simulink model "vehicleVariantsLabel"  (R2020a)
settings: Solver=VariableStepAuto  StartTime=0.0  StopTime=30  FixedStep=Ts  RelTol=1e-3
model workspace: external: MAT-File data.mat (data not in the file)
values from neighbouring files (symbols this model uses):
  fsw = 9000    [data.mat]
  ID_MAP = [-123.486133396 -123.486133396 -123.486133396 -123.486133396 -123.486133396 -123.486133396 -123.486133396 -123.486133396 -123.486133396 -123.486133396 -123.486133396 -123.486133396 ... (280623 elements, 161x83x21)]    [data.mat]
  IQ_MAP = [-339.521551914 -339.521551914 -339.521551914 -339.521551914 -339.521551914 -339.521551914 -339.521551914 -339.521551914 -339.521551914 -339.521551914 -339.521551914 -339.521551914 ... (280623 elements, 161x83x21)]    [data.mat]
  Ki_v = 70    [data.mat]
  Kp_v = 150    [data.mat]
  Ld = 0.00024368    [data.mat]
  Lq = 0.00029758    [data.mat]
  motorOn = 1    [data.mat]
  p = 8    [data.mat]
  Pmax = 35000    [data.mat]
  psim = 0.04366    [data.mat]
  recumax = -50    [data.mat]
  RPM_VECT = [0 100 200 300 400 500 600 700 800 900 1000 1100 ... (161 elements, 1x161)]    [data.mat]
  rreifen = 0.3237    [data.mat]
  Tmax = 205    [data.mat]
  TQ_VECT = [-205 -200 -195 -190 -185 -180 -175 -170 -165 -160 -155 -150 ... (83 elements, 1x83)]    [data.mat]
  Ts = 5e-05    [data.mat]
  Tsi = 5e-05    [data.mat]
  Tso = 0.0005    [data.mat]
  VDC_VECT = [300 305 310 315 320 325 330 335 340 345 350 355 ... (21 elements, 1x21)]    [data.mat]
  Vnom = 325    [data.mat]
undefined symbols (not defined in the file or in its folder): DiscIntNeverNeededParam, sigbuilder_block
libraries: fl_lib x42, nesl_utility x20, ee_lib x8, simulink x2, eeTransforms x2, eeDiscretePi x1, eePmsmCurrentController x1, eePwmGeneratorTwoLevel x1
(part 1 of 2)
settings Model: SimulationMode=accelerator  OrderedModelArguments=off  Creator=ftutschk  LastModifiedBy=ftutschk
settings DataIOCC: SaveOutput=off  DSMLogging=off  SaveTime=off  ReturnWorkspaceOutputs=off
settings DebuggingCC: ArithmeticOperatorsInVariantConditions=warning
settings SFSimCC: SimUseLocalCustomCode=off  CustomCodeUndefinedFunction=UseInterfaceOnly
settings RTWCC: RTWUseLocalCustomCode=off

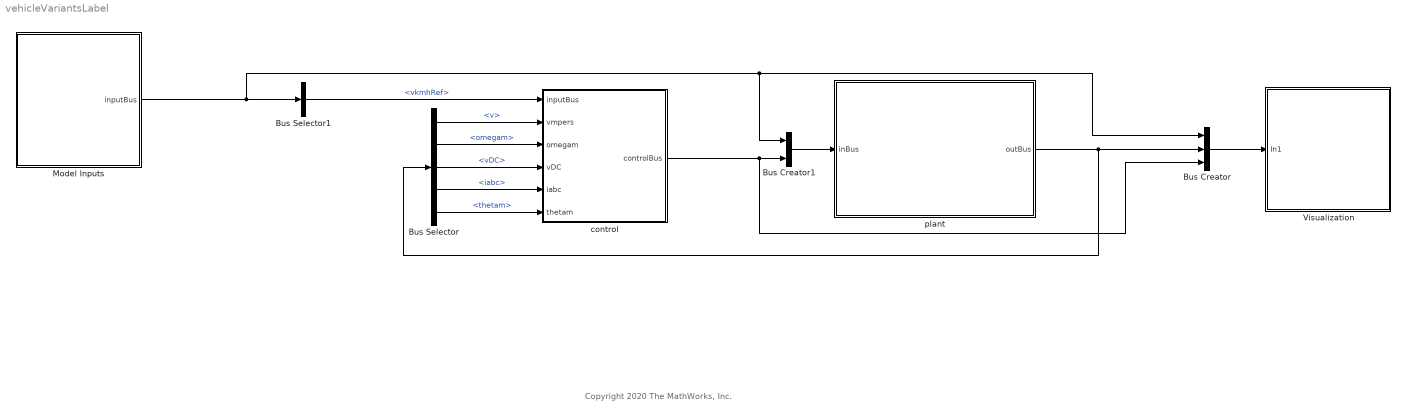
== system vehicleVariantsLabel ==
  note: Copyright 2020 The MathWorks, Inc.
  Bus Creator : BusCreator  Inputs=3
  Bus Creator1 : BusCreator  Inputs=2
  Bus Selector : BusSelector  OutputSignals=v,omegam,vDC,iabc,thetam
  Bus Selector1 : BusSelector  OutputSignals=vkmhRef
  Model Inputs : Subsystem  Variant=on  VariantControlMode=Label  LabelModeActiveChoice=Signal Builder
  Visualization : Subsystem  SystemSampleTime=1e-3
  control : Subsystem  VariantControl=Variant
  plant : Subsystem
  wires:
  plant/1(outBus) -> Bus Creator/2, Bus Selector/1
  Bus Selector1/1 -> control/1(inputBus)  "<vkmhRef>"
  Bus Creator1/1 -> plant/1(inBus)
  Bus Selector/2 -> control/3(omegam)  "<omegam>"
  control/1(controlBus) -> Bus Creator/3, Bus Creator1/2
  Bus Selector/1 -> control/2(vmpers)  "<v>"
  Bus Selector/5 -> control/6(thetam)  "<thetam>"
  Model Inputs/1(inputBus) -> Bus Creator/1, Bus Creator1/1, Bus Selector1/1
  Bus Selector/4 -> control/5(iabc)  "<iabc>"
  Bus Selector/3 -> control/4(vDC)  "<vDC>"
  Bus Creator/1 -> Visualization/1(In1)

== system vehicleVariantsLabel/Model Inputs ==
  Signal Builder : Subsystem  VariantControl=Signal Builder
      mask Display: text(0.5,0.5,  '{\fontsize{12} \bfSignal Builder}', 'texmode','on','horizontalAlignment', 'center');
  other : Subsystem  VariantControl=other
      mask Display: text(0.5,0.5,  '{\fontsize{12} \bfother}', 'texmode','on','horizontalAlignment', 'center');
  inputBus : Outport  VectorParamsAs1DForOutWhenUnconnected=off

== system vehicleVariantsLabel/Visualization ==
  In1 : Inport
  Bus Selector : BusSelector  OutputSignals=carBus.iabc,carBus.vabc,carBus.v,inputBus.vkmhRef,controlBus.trq_cmd,controlBus.trqLim,controlBus.fricTrq_cmd,controlBus.eTrq_cmd,carBus.trqMech,carBus.vDC,controlBus.vdq
  Gain : Gain  Gain=3.6
  Gain1 : Gain  Gain=1/sqrt(3)
  Mux3 : Mux  Inputs=2
  Mux4 : Mux  Inputs=5
  Mux5 : Mux  Inputs=2
  Rate Transition2 : RateTransition
  Scope : Scope  NumInputPorts=5
  wires:
  Bus Selector/9 -> Mux4/3  "<trqMech>"
  Bus Selector/3 -> Gain/1  "<v>"
  Bus Selector/4 -> Rate Transition2/1  "<vkmhRef>"
  Gain/1 -> Mux3/1  "vkm_h"
  Bus Selector/5 -> Mux4/1  "<trq_cmd>"
  Bus Selector/6 -> Mux4/2  "<trqLim>"
  Bus Selector/10 -> Gain1/1  "<vDC>"
  Gain1/1 -> Mux5/1
  Bus Selector/11 -> Mux5/2  "<vdq>"
  Bus Selector/7 -> Mux4/4  "<fricTrq_cmd>"
  Bus Selector/8 -> Mux4/5  "<eTrq_cmd>"
  Bus Selector/1 -> Scope/1  "<iabc>"
  Bus Selector/2 -> Scope/2  "<vabc>"
  Mux3/1 -> Scope/3
  Mux4/1 -> Scope/4
  Mux5/1 -> Scope/5
  Rate Transition2/1 -> Mux3/2
  In1/1 -> Bus Selector/1

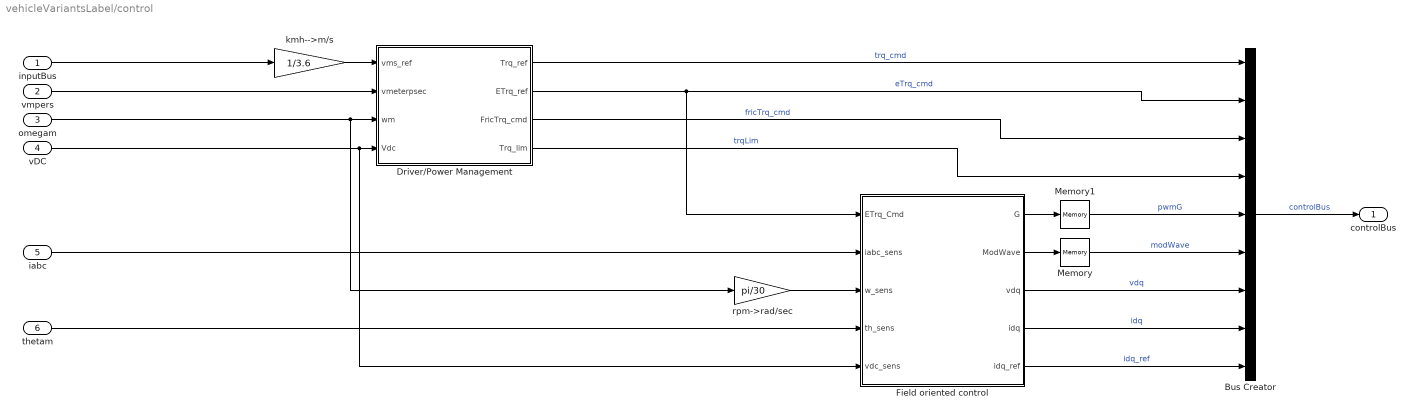
== system vehicleVariantsLabel/control ==
  inputBus : Inport
  vmpers : Inport  Port=2
  omegam : Inport  Port=3
  vDC : Inport  Port=4
  iabc : Inport  Port=5
  thetam : Inport  Port=6
  Bus Creator : BusCreator  Inputs=9
  Driver/Power Management : Subsystem
  "Field oriented control " : Subsystem  VariantControl=VAR_ANTRIEB_HECK
  Memory : Memory
  Memory1 : Memory
  kmh-->m/s : Gain  Gain=1/3.6
  rpm->rad/sec : Gain  Gain=pi/30
  controlBus : Outport  VectorParamsAs1DForOutWhenUnconnected=off
  wires:
  vmpers/1 -> Driver/Power Management/2(vmeterpsec)
  kmh-->m/s/1 -> Driver/Power Management/1(vms_ref)
  Driver/Power Management/1(Trq_ref) -> Bus Creator/1  "trq_cmd"
  Driver/Power Management/3(FricTrq_cmd) -> Bus Creator/3  "fricTrq_cmd"
  Driver/Power Management/4(Trq_lim) -> Bus Creator/4  "trqLim"
  Driver/Power Management/2(ETrq_ref) -> "Field oriented control "/1(ETrq_Cmd), Bus Creator/2  "eTrq_cmd"
  omegam/1 -> rpm->rad/sec/1, Driver/Power Management/3(wm)
  vDC/1 -> "Field oriented control "/5(vdc_sens), Driver/Power Management/4(Vdc)
  inputBus/1 -> kmh-->m/s/1
  Memory1/1 -> Bus Creator/5  "pwmG"
  Bus Creator/1 -> controlBus/1  "controlBus"
  Memory/1 -> Bus Creator/6  "modWave"
  iabc/1 -> "Field oriented control "/2(iabc_sens)
  rpm->rad/sec/1 -> "Field oriented control "/3(w_sens)
  thetam/1 -> "Field oriented control "/4(th_sens)
  "Field oriented control "/1(G) -> Memory1/1
  "Field oriented control "/2(ModWave) -> Memory/1
  "Field oriented control "/3(vdq) -> Bus Creator/7  "vdq"
  "Field oriented control "/4(idq) -> Bus Creator/8  "idq"
  "Field oriented control "/5(idq_ref) -> Bus Creator/9  "idq_ref"

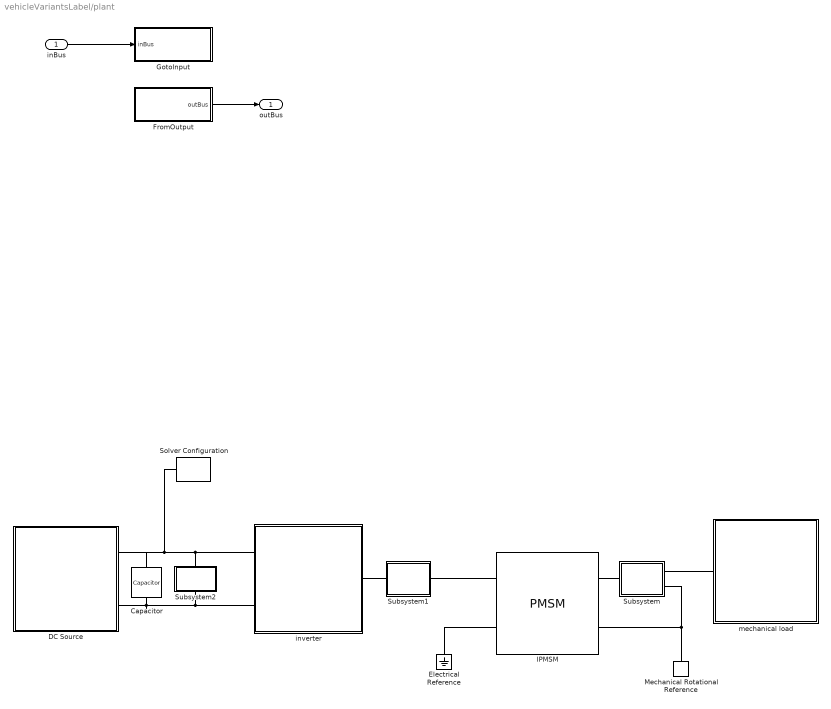
== system vehicleVariantsLabel/plant ==
  inBus : Inport
  Capacitor : fl_lib/Electrical/Electrical Elements/Capacitor  c=1e-3 F  r=0 Ohm  g=0 1/Ohm  i_specify=off  i_priority=None  i=0 A  i_nominal_specify=off  i_nominal_unit=A  i_nominal_value=1  v_specify=off  v_priority=None  v=0 V  v_nominal_specify=off  v_nominal_unit=V  v_nominal_value=1  vc_specify=on  vc_priority=High  vc=Vnom V  vc_nominal_specify=off  vc_nominal_unit=V  vc_nominal_value=1
  DC Source : Subsystem  Variant=on  VariantControlMode=Label  LabelModeActiveChoice=DC ideal
  Electrical Reference : fl_lib/Electrical/Electrical Elements/Electrical Reference
  FromOutput : Subsystem
  GotoInput : Subsystem
  IPMSM : ee_lib/Electromechanical/Permanent Magnet/PMSM  winding_type=ee.enum.statorconnection.wye  machine_param=ee.enum.pmsm.parameterization.constant  nPolePairs=p  pmflux_param=1  pm_flux_linkage=psim Wb  torque_constant=0.18 N*m/A  back_emf_constant=0.18 V/(rad/s)  stator_param=ee.enum.statorparam.LdLqL0  Ld=Ld H  Lq=Lq H  idVec=[-200, 0, 200] A  iqVec=[-200, 0, 200] A  LdMatrix=0.0002 * ones(3, 3) H  LqMatrix=0.0002 * ones(3, 3) H  PmMatrix=0.1 * ones(3, 3) Wb  ktMatrix=0.18 * ones(3, 3) N*m/A  keMatrix=0.18 * ones(3, 3) V/(rad/s)  L0=L0 H  Ls=0.0002 H  Lm=0.00002 H  Ms=0.00002 H  Rs=Rs Ohm  zero_sequence=ee.enum.park.zerosequence.exclude  J=0 kg*m^2  lam=0 N*m/(rad/s)  axes_param=ee.enum.rotorangle.qaxis  i_d_specify=off  i_d_priority=None  i_d=0 A  i_d_nominal_specify=off  i_d_nominal_unit=A  i_d_nominal_value=1  i_q_specify=off  i_q_priority=None  i_q=0 A  i_q_nominal_specify=off  i_q_nominal_unit=A  i_q_nominal_value=1  torque_specify=off  torque_priority=None  torque=0 N*m  torque_nominal_specify=off  torque_nominal_unit=N*m  torque_nominal_value=1  angular_velocity_specify=on  angular_velocity_priority=None  angular_velocity=0 rpm  angular_velocity_nominal_specify=off  angular_velocity_nominal_unit=rpm  angular_velocity_nominal_value=1  angular_position_specify=on  angular_position_priority=High  angular_position=0 rad  angular_position_nominal_specify=off  angular_position_nominal_unit=deg  angular_position_nominal_value=1  loss_param=ee.enum.ironloss.none  losses_oc=[0, 0, 0] W  losses_sc=[0, 0, 0] W  f_losses=60 Hz  Isc_losses=95 A  Tmeas=298.15 K  alpha=3.93e-3 1/K  alpha_flux=-0.001 1/K  stator_thermal_mass=100 J/K  rotor_thermal_mass=200 J/K  Rm_percent_rotor=90  Rd_percent_rotor=30  temperatureA_specify=off  temperatureA_priority=High  temperatureA=25 degC  temperatureA_nominal_specify=off  temperatureA_nominal_unit=degC  temperatureA_nominal_value=1  temperatureB_specify=off  temperatureB_priority=High  temperatureB=25 degC  temperatureB_nominal_specify=off  temperatureB_nominal_unit=degC  temperatureB_nominal_value=1  temperatureC_specify=off  temperatureC_priority=High  temperatureC=25 degC  temperatureC_nominal_specify=off  temperatureC_nominal_unit=degC  temperatureC_nominal_value=1  temperatureR_specify=off  temperatureR_priority=High  temperatureR=25 degC  temperatureR_nominal_specify=off  temperatureR_nominal_unit=degC  temperatureR_nominal_value=1
      settings: InternalSimscapePortConfiguration="{\"Bottom\":[],\"Left\":[{\"id\":\"N\",\"label\":\"~\",\"type\":\"foundation.electrical.three_phase\"},{\"id\":\"n\",\"label\":\"n\",\"type\":\"foundation.electrical.electrical\"}],\"Right\":[{\"id\":\"R\",\"label\":\"R\",\"type\":\"foundation.mechanical.rotational.rotational\"},{\"id\":\"C\",\"label\":\"C\",\"type\":\"foundation.mechanical.rotational.rotational\"}],\"Top\":[]}"
  Mechanical Rotational Reference : fl_lib/Mechanical/Rotational Elements/Mechanical Rotational Reference
  Solver Configuration : nesl_utility/Solver Configuration  PhysicalDomain=network_engine_domain  SubClassName=solver  LeftPortType=input  RightPortType=generic  Tones=[]  Harmonics=[]  SimulateNoise=off  Profile=off  UseLocalSampling=off  EnableSwitchedLinearOptims=on  FrequencyDomain=off  UseCCode=off  RelTol=0.001  AbsTol=1e-06  MinStep=1e-09  ToWorkspace=off  RevertToSquareIcSolve=off  NumHomotopyIterations=100  PhasorMode=off  PhasorModeNumHarmonics=1  DoDC=off  ResidualTolerance=1e-09  UseLocalSolver=on  LocalSolverChoice=NE_BACKWARD_EULER_ADVANCER  LocalSolverSampleTime=Ts  DoFixedCost=on  MaxNonlinIter=5  MaxModeIter=2  LinearAlgebra=Sparse  EquationFormulation=NE_TIME_EF  DelaysMemoryBudget=2048  AutomaticFiltering=on  FilteringTimeConstant=0.001  PartitionStorageMethod=AS_NEEDED  PartitionMemoryBudget=1024  PartitionMethod=FAST
  Subsystem : Subsystem
      mask Display: text(0.5,0.5, '{\fontsize{14} Sensor}', 'texmode','on','horizontalAlignment', 'center');
  Subsystem1 : Subsystem
      mask Display: text(0.5,0.5, '{\fontsize{14} Sensor}', 'texmode','on','horizontalAlignment', 'center');
  Subsystem2 : Subsystem
      mask Display: text(0.5,0.5, '{\fontsize{14} Sensor}', 'texmode','on','horizontalAlignment', 'center');
  inverter : Subsystem  Variant=on  VariantControlMode=Label  LabelModeActiveChoice=average voltage inverter
  mechanical load : Subsystem  Variant=on  VariantControlMode=Label  LabelModeActiveChoice=load1
  outBus : Outport  VectorParamsAs1DForOutWhenUnconnected=off
  wires:
  FromOutput/1(outBus) -> outBus/1
  inBus/1 -> GotoInput/1(inBus)
  connections:
  Subsystem/RConn1 -- mechanical load/LConn1
  IPMSM/RConn2 -- Mechanical Rotational Reference/LConn1 -- Subsystem/RConn2
  IPMSM/RConn1 -- Subsystem/LConn1
  Solver Configuration/RConn1 -- Capacitor/LConn1 -- DC Source/RConn1 -- inverter/LConn1 -- Subsystem2/LConn1
  DC Source/RConn2 -- Capacitor/RConn1 -- inverter/LConn2 -- Subsystem2/RConn1
  Electrical Reference/LConn1 -- IPMSM/LConn2
  Subsystem1/LConn1 -- inverter/RConn1
  Subsystem1/RConn1 -- IPMSM/LConn1

== system vehicleVariantsLabel/Model Inputs/Signal Builder ==
  Bus Creator1 : BusCreator  Inputs=3
  Signal Builder : Subsystem  Tag=STV Subsys  LoadFcn=sigbuilder_block('load');  StartFcn=sigbuilder_block('start');  StopFcn=sigbuilder_block('stop');  ClipboardFcn=sigbuilder_block('clipboard');  mask(Sigbuilder block){tuvar=[0:10]}
      mask help: Simulink:masks:SigbuilderBlock_MD
      mask init:
      | if ~strcmp(get_param(bdroot(gcbh),'SimulationStatus'),'stopped') tuvar = sigbuilder_block('maskInit'); end
      settings: CopyFcn=sigbuilder_block('copy');  DeleteFcn=sigbuilder_block('delete');  ModelCloseFcn=sigbuilder_block('modelClose');  PreSaveFcn=sigbuilder_block('preSave');  PauseFcn=sigbuilder_block('pause');  ContinueFcn=sigbuilder_block('continue');  NameChangeFcn=sigbuilder_block('namechange');  OpenFcn=sigbuilder_block('open',[52.5 136.5 1247.25 609.75 ]);  CloseFcn=sigbuilder_block('close');
      mask Display: plot(0, 0, 100, 100,[2, 2, 32, 32, 2], [68, 8, 8, 68, 68],[32, 2], [38, 38], [32, 19, 2],[53, 60, 44], [32, 17, 17, 2],[16, 16, 31, 31]);txt = getActiveGroup(gcbh);text(2, 100, txt,'verticalAlignment', 'top');
  deg-->rad : Gain  Gain=pi/180
  inputBus : Outport  VectorParamsAs1DForOutWhenUnconnected=off
  wires:
  Signal Builder/2(grade[deg]) -> deg-->rad/1
  Signal Builder/1(v [km/h]) -> Bus Creator1/1  "vkmhRef"
  Bus Creator1/1 -> inputBus/1  "inputBus"
  Signal Builder/3(vWind [m/s]) -> Bus Creator1/3  "vWind"
  deg-->rad/1 -> Bus Creator1/2  "grade"

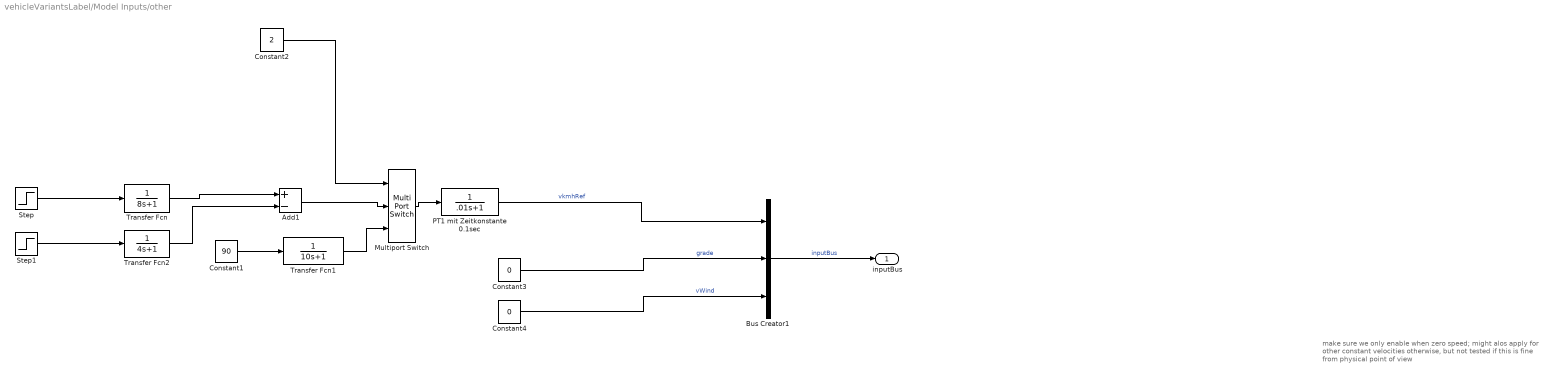
== system vehicleVariantsLabel/Model Inputs/other ==
  note: make sure we only enable when zero speed; might alos apply
      |  for other constant velocities otherwise, but not tested if this is
      |  fine from physical point of view
  Add1 : Sum  Inputs=+-
  Bus Creator1 : BusCreator  Inputs=3
  Constant1 : Constant  Value=90
  Constant2 : Constant  Value=2
  Constant3 : Constant  Value=0
  Constant4 : Constant  Value=0
  Multiport Switch : MultiPortSwitch  Inputs=2
  PT1 mit Zeitkonstante 0.1sec : TransferFcn  Denominator=[.01 1]
  Step : Step  After=25  SampleTime=0
  Step1 : Step  Time=10  After=10  SampleTime=0
  Transfer Fcn : TransferFcn  Denominator=[8 1]
  Transfer Fcn1 : TransferFcn  Denominator=[10 1]
  Transfer Fcn2 : TransferFcn  Denominator=[4 1]
  inputBus : Outport  VectorParamsAs1DForOutWhenUnconnected=off
  wires:
  Multiport Switch/1 -> PT1 mit Zeitkonstante 0.1sec/1
  Constant1/1 -> Transfer Fcn1/1
  Step/1 -> Transfer Fcn/1
  Transfer Fcn1/1 -> Multiport Switch/3
  Step1/1 -> Transfer Fcn2/1
  Add1/1 -> Multiport Switch/2
  Transfer Fcn/1 -> Add1/1
  Transfer Fcn2/1 -> Add1/2
  Constant2/1 -> Multiport Switch/1
  Bus Creator1/1 -> inputBus/1  "inputBus"
  PT1 mit Zeitkonstante 0.1sec/1 -> Bus Creator1/1  "vkmhRef"
  Constant3/1 -> Bus Creator1/2  "grade"
  Constant4/1 -> Bus Creator1/3  "vWind"

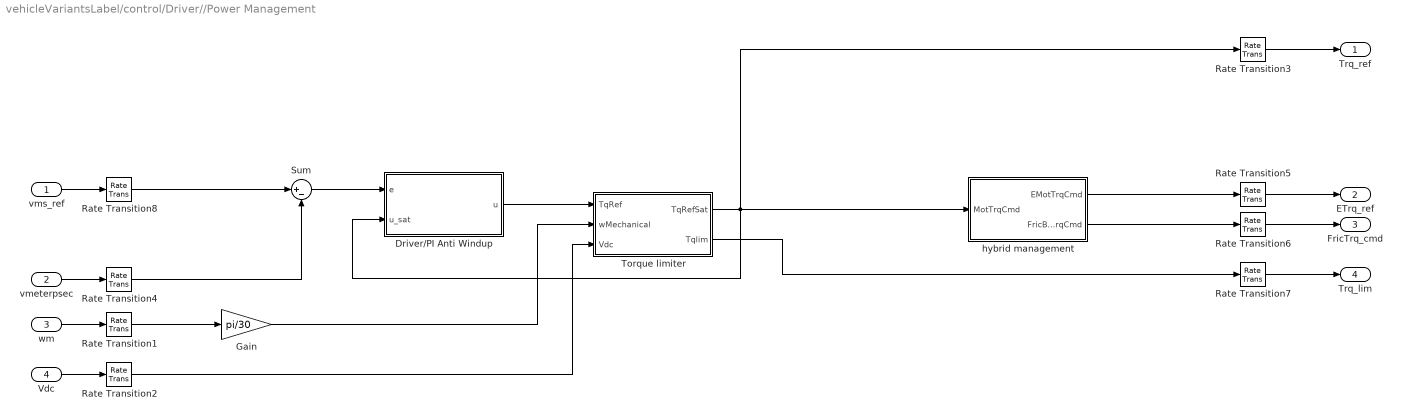
== system vehicleVariantsLabel/control/Driver//Power Management ==
  vms_ref : Inport
  vmeterpsec : Inport  Port=2
  wm : Inport  Port=3
  Vdc : Inport  Port=4
  Driver/PI Anti Windup : Subsystem
  Gain : Gain  Gain=pi/30
  Rate Transition{1..2,4,8} (4 alike) : RateTransition  OutPortSampleTime=Tso
  Rate Transition{3,5..7} (4 alike) : RateTransition
  Sum : Sum  Inputs=|+-
  Torque limiter : Subsystem
  hybrid management : Subsystem  VariantControl=VAR_ANTRIEB_HECK
  Trq_ref : Outport  VectorParamsAs1DForOutWhenUnconnected=off
  ETrq_ref : Outport  Port=2  VectorParamsAs1DForOutWhenUnconnected=off
  FricTrq_cmd : Outport  Port=3  VectorParamsAs1DForOutWhenUnconnected=off
  Trq_lim : Outport  Port=4  VectorParamsAs1DForOutWhenUnconnected=off
  wires:
  wm/1 -> Rate Transition1/1
  Torque limiter/2(Tqlim) -> Rate Transition7/1
  vms_ref/1 -> Rate Transition8/1
  Torque limiter/1(TqRefSat) -> hybrid management/1(MotTrqCmd), Rate Transition3/1, Driver/PI Anti Windup/2(u_sat)
  Rate Transition8/1 -> Sum/1
  Vdc/1 -> Rate Transition2/1
  Rate Transition1/1 -> Gain/1
  Rate Transition2/1 -> Torque limiter/3(Vdc)
  vmeterpsec/1 -> Rate Transition4/1
  Rate Transition4/1 -> Sum/2
  Sum/1 -> Driver/PI Anti Windup/1(e)
  Driver/PI Anti Windup/1(u) -> Torque limiter/1(TqRef)
  Rate Transition3/1 -> Trq_ref/1
  Rate Transition5/1 -> ETrq_ref/1
  Rate Transition6/1 -> FricTrq_cmd/1
  Rate Transition7/1 -> Trq_lim/1
  Gain/1 -> Torque limiter/2(wMechanical)
  hybrid management/1(EMotTrqCmd) -> Rate Transition5/1
  hybrid management/2("FricBrakeTrqCmd ") -> Rate Transition6/1

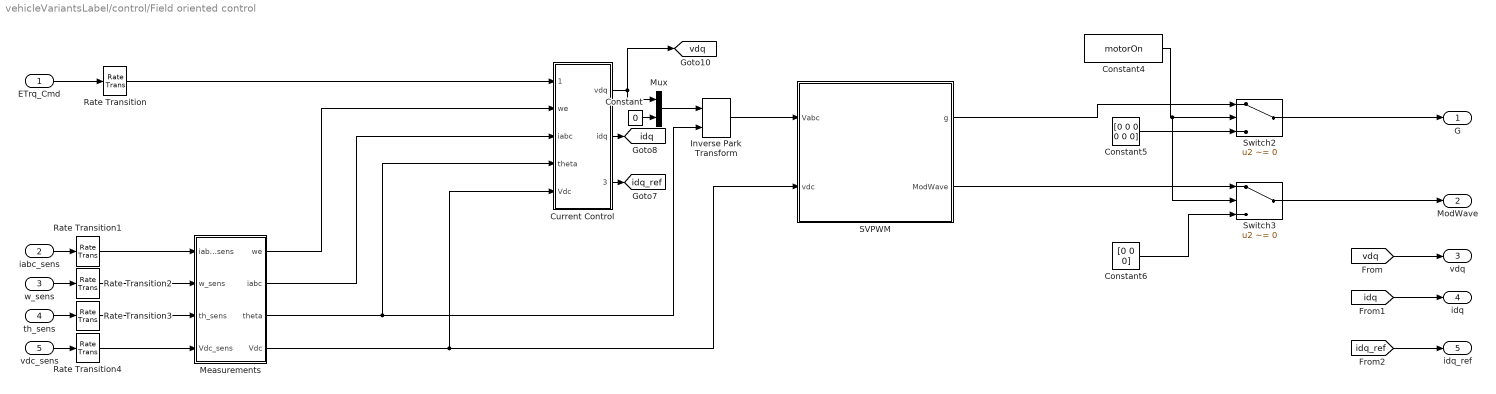
== system vehicleVariantsLabel/control/Field oriented control  ==
  ETrq_Cmd : Inport
  iabc_sens : Inport  Port=2
  w_sens : Inport  Port=3
  th_sens : Inport  Port=4
  vdc_sens : Inport  Port=5
  Constant : Constant  Value=0  SampleTime=-1
  Constant4 : Constant  Value=motorOn
  Constant5 : Constant  Value=[0 0 0 0 0 0]
  Constant6 : Constant  Value=[0 0 0]
  Current Control : Subsystem
  Inverse Park Transform : eeTransforms/Inverse Park Transform  AxisAlignment=Q-axis  PowerInvariant=off
  Measurements : Subsystem
  Mux : Mux  Inputs=2
  Rate Transition{,1..4} (5 alike) : RateTransition  OutPortSampleTime=Tsi
  SVPWM : Subsystem  Tag=noUIvariant  Variant=on  VariantControlMode=Label  LabelModeActiveChoice=Variant
  Switch2 : Switch  Criteria=u2 ~= 0
  Switch3 : Switch  Criteria=u2 ~= 0
  G : Outport  VectorParamsAs1DForOutWhenUnconnected=off
  ModWave : Outport  Port=2  VectorParamsAs1DForOutWhenUnconnected=off
  vdq : Outport  Port=3  VectorParamsAs1DForOutWhenUnconnected=off
  idq : Outport  Port=4  VectorParamsAs1DForOutWhenUnconnected=off
  idq_ref : Outport  Port=5  VectorParamsAs1DForOutWhenUnconnected=off
  tag scope: idq=global, idq_ref=global, vdq=global
  wires:
  Current Control/3(idq_ref) -> [idq_ref]
  ETrq_Cmd/1 -> Rate Transition/1
  Measurements/3(theta) -> Current Control/4(theta), Inverse Park Transform/2
  Constant/1 -> Mux/2
  Mux/1 -> Inverse Park Transform/1
  Current Control/2(idq) -> [idq]
  Measurements/1(we) -> Current Control/2(we)
  Measurements/4(Vdc) -> SVPWM/2(vdc), Current Control/5(Vdc)
  vdc_sens/1 -> Rate Transition4/1
  th_sens/1 -> Rate Transition3/1
  w_sens/1 -> Rate Transition2/1
  iabc_sens/1 -> Rate Transition1/1
  Measurements/2(iabc) -> Current Control/3(iabc)
  Current Control/1(vdq) -> [vdq], Mux/1
  Rate Transition/1 -> Current Control/1(Tq_ref)
  Rate Transition1/1 -> Measurements/1(iabc_sens)
  Rate Transition2/1 -> Measurements/2(w_sens)
  Rate Transition3/1 -> Measurements/3(th_sens)
  Rate Transition4/1 -> Measurements/4(Vdc_sens)
  Inverse Park Transform/1 -> SVPWM/1(Vabc)
  Constant6/1 -> Switch3/3
  Switch3/1 -> ModWave/1
  Constant5/1 -> Switch2/3
  Constant4/1 -> Switch3/2, Switch2/2
  Switch2/1 -> G/1
  SVPWM/1(g) -> Switch2/1
  SVPWM/2(ModWave) -> Switch3/1
  [vdq] -> vdq/1
  [idq] -> idq/1
  [idq_ref] -> idq_ref/1

== system vehicleVariantsLabel/plant/DC Source ==
  DC ideal : Subsystem  VariantControl=DC ideal
  battery : Subsystem  VariantControl=battery
  + : PMIOPort  Side=Right
  - : PMIOPort  Port=2  Side=Right

== system vehicleVariantsLabel/plant/FromOutput ==
  Bus Creator : BusCreator  Inputs=8
  outBus : Outport  VectorParamsAs1DForOutWhenUnconnected=off
  wires:
  [v] -> Bus Creator/1  "v"
  [omegam] -> Bus Creator/2  "omegam"
  [thetam] -> Bus Creator/3  "thetam"
  Bus Creator/1 -> outBus/1  "carBus"
  [Tmech] -> Bus Creator/4  "trqMech"
  [iabc] -> Bus Creator/5  "iabc"
  [vabc] -> Bus Creator/6  "vabc"
  [vDC] -> Bus Creator/7  "vDC"
  [SOC] -> Bus Creator/8  "SOC"

== system vehicleVariantsLabel/plant/GotoInput ==
  inBus : Inport
  Bus Selector : BusSelector  OutputSignals=controlBus.pwmG,controlBus.modWave,controlBus.fricTrq_cmd
  tag scope: FricTrq_cmd=global, G=global, modwave=global
  wires:
  inBus/1 -> Bus Selector/1
  Bus Selector/1 -> [G]  "<pwmG>"
  Bus Selector/2 -> [modwave]  "<modWave>"
  Bus Selector/3 -> [FricTrq_cmd]  "<fricTrq_cmd>"

== system vehicleVariantsLabel/plant/Subsystem ==
  Ideal Rotational Motion Sensor : fl_lib/Mechanical/Mechanical Sensors/Ideal Rotational Motion Sensor  wrap_angle=simscape.enum.onoff.off  offset=0 rad
  Ideal Torque Sensor : fl_lib/Mechanical/Mechanical Sensors/Ideal Torque Sensor
  PS-Simulink Converter : nesl_utility/PS-Simulink Converter  PhysicalDomain=network_engine_domain  SubClassName=ps_output  LeftPortType=input  RightPortType=output  PseudoPeriodic=off  Frequencies=[]  Unit=rpm  AffineConversion=off
  PS-Simulink Converter1 : nesl_utility/PS-Simulink Converter  PhysicalDomain=network_engine_domain  SubClassName=ps_output  LeftPortType=input  RightPortType=output  PseudoPeriodic=off  Frequencies=[]  Unit=N*m  AffineConversion=off
  PS-Simulink Converter2 : nesl_utility/PS-Simulink Converter  PhysicalDomain=network_engine_domain  SubClassName=ps_output  LeftPortType=input  RightPortType=output  PseudoPeriodic=off  Frequencies=[]  Unit=rad  AffineConversion=off
  R2 : PMIOPort  Side=Right
  R1 : PMIOPort  Port=2  Side=Left
  C : PMIOPort  Port=3  Side=Right
  tag scope: Tmech=global, omegam=global, thetam=global
  wires:
  PS-Simulink Converter/1 -> [omegam]
  PS-Simulink Converter1/1 -> [Tmech]
  PS-Simulink Converter2/1 -> [thetam]
  connections:
  Ideal Rotational Motion Sensor/RConn2 -- PS-Simulink Converter/LConn1
  R1/RConn1 -- Ideal Torque Sensor/LConn1
  Ideal Rotational Motion Sensor/LConn1 -- R2/RConn1 -- Ideal Torque Sensor/RConn1
  Ideal Torque Sensor/RConn2 -- PS-Simulink Converter1/LConn1
  Ideal Rotational Motion Sensor/RConn3 -- PS-Simulink Converter2/LConn1
  Ideal Rotational Motion Sensor/RConn1 -- C/RConn1

== system vehicleVariantsLabel/plant/Subsystem1 ==
  Current Sensor (Three-Phase) : ee_lib/Sensors & Transducers/Current Sensor (Three-Phase)
  Current and Voltage Sensor (Three-Phase) : ee_lib/Sensors & Transducers/Current and Voltage Sensor (Three-Phase)  vMeasurementType=ee.enum.vmeasurement.lg  outputUnit=ee.enum.unit.si  SRated=100e6 V*A  VRated=24e3 V  I_specify=off  I_priority=None  I=[ 0 0 0 ] A  I_nominal_specify=off  I_nominal_unit=A  I_nominal_value=1  V_specify=off  V_priority=None  V=[ 0 0 0 ] V  V_nominal_specify=off  V_nominal_unit=V  V_nominal_value=1
      settings: SourceProductBaseCode=PS  InternalSimscapePortConfiguration="{\"Bottom\":[],\"Left\":[{\"id\":\"N1\",\"label\":\"~1\",\"type\":\"foundation.electrical.three_phase\"}],\"Right\":[{\"id\":\"V_output\",\"label\":\"V\",\"type\":\"output\"},{\"id\":\"I_output\",\"label\":\"I\",\"type\":\"output\"},{\"id\":\"N2\",\"label\":\"~2\",\"type\":\"foundation.electrical.three_phase\"}],\"Top\":[]}"
  PS-Simulink Converter : nesl_utility/PS-Simulink Converter  PhysicalDomain=network_engine_domain  SubClassName=ps_output  LeftPortType=input  RightPortType=output  PseudoPeriodic=off  Frequencies=[]  Unit=inherit  AffineConversion=off
  PS-Simulink Converter1 : nesl_utility/PS-Simulink Converter  PhysicalDomain=network_engine_domain  SubClassName=ps_output  LeftPortType=input  RightPortType=output  PseudoPeriodic=off  Frequencies=[]  Unit=inherit  AffineConversion=off
  PS-Simulink Converter2 : nesl_utility/PS-Simulink Converter  PhysicalDomain=network_engine_domain  SubClassName=ps_output  LeftPortType=input  RightPortType=output  PseudoPeriodic=off  Frequencies=[]  Unit=inherit  AffineConversion=off
  Scope : Scope
  ~2 : PMIOPort  Side=Right
  ~1 : PMIOPort  Port=2  Side=Left
  tag scope: iabc=global, vabc=global
  wires:
  PS-Simulink Converter1/1 -> [iabc]
  PS-Simulink Converter/1 -> [vabc]
  PS-Simulink Converter2/1 -> Scope/1
  connections:
  Current and Voltage Sensor (Three-Phase)/LConn1 -- ~1/RConn1
  Current and Voltage Sensor (Three-Phase)/RConn1 -- PS-Simulink Converter/LConn1
  Current and Voltage Sensor (Three-Phase)/RConn2 -- PS-Simulink Converter1/LConn1
  Current Sensor (Three-Phase)/LConn1 -- Current and Voltage Sensor (Three-Phase)/RConn3
  Current Sensor (Three-Phase)/RConn2 -- ~2/RConn1
  Current Sensor (Three-Phase)/RConn1 -- PS-Simulink Converter2/LConn1

== system vehicleVariantsLabel/plant/Subsystem2 ==
  PS-Simulink Converter : nesl_utility/PS-Simulink Converter  PhysicalDomain=network_engine_domain  SubClassName=ps_output  LeftPortType=input  RightPortType=output  PseudoPeriodic=off  Frequencies=[]  Unit=inherit  AffineConversion=off
  Voltage Sensor : fl_lib/Electrical/Electrical Sensors/Voltage Sensor
  Conn1 : PMIOPort  Side=Left
  Conn2 : PMIOPort  Port=2  Side=Right
  tag scope: vDC=global
  wires:
  PS-Simulink Converter/1 -> [vDC]
  connections:
  Conn2/RConn1 -- Voltage Sensor/RConn2
  Voltage Sensor/RConn1 -- PS-Simulink Converter/LConn1
  Voltage Sensor/LConn1 -- Conn1/RConn1

== system vehicleVariantsLabel/plant/inverter ==
  Average Voltage inverter : Subsystem  VariantControl=average voltage inverter
  ideal inverter : Subsystem  VariantControl=ideal inverter
  + : PMIOPort  Side=Left
  - : PMIOPort  Port=2  Side=Left
  ~2 : PMIOPort  Port=3  Side=Right

== system vehicleVariantsLabel/plant/mechanical load ==
  load1 : Subsystem  VariantControl=load1
  load2 : Subsystem  VariantControl=load2
  R : PMIOPort  Side=Left

== system vehicleVariantsLabel/Model Inputs/Signal Builder/Signal Builder ==
  Demux : Demux  Tag=STV Demux  Outputs=3
      settings: DisplayOption=none
  FromWs : FromWorkspace  Tag=STV FromWs  VariableName=tuvar
      SigBuilderData=|
      | common.afterFinalStr = 'Extrapolate'
      | common.sampleTime = 0
      | dataSet(1).timeRange = [0 5]
      | dataSet(1).name = 'Group 1'
      | dataSet(2).timeRange = [0 15]
      | dataSet(2).name = 'Group 2'
      | dataSet(3).timeRange = [0 10]
      | dataSet(3).name = 'Group 3'
      | dataSet(4).timeRange = [0 10]
      | dataSet(4).name = 'Group 4'
      | dataSet(5).timeRange = [0 12]
      | dataSet(5).name = 'Group 5'
      | dataSet(6).timeRange = [0 30]
      | dataSet(6).name = 'Group 6'
      | sbobj.Groups(1).Name = 'Group 1'
      | sbobj.Groups(1).Signals(1).Name = 'v [km/h]'
      | sbobj.Groups(1).Signals(1).XData = [0 3 5]
      | sbobj.Groups(1).Signals(1).YData = [0 30 30]
      | sbobj.Groups(1).Signals(2).Name = 'grade[deg]'
      | sbobj.Groups(1).Signals(2).XData = [0 5]
      | sbobj.Groups(1).Signals(2).YData = [0 0]
      | sbobj.Groups(1).Signals(3).Name = 'vWind [m/s]'
      | sbobj.Groups(1).Signals(3).XData = [0 5]
      | sbobj.Groups(1).Signals(3).YData = [0 0]
      | sbobj.Groups(1).TimeRange = [0 5]
      | sbobj.Groups(2).Name = 'Group 2'
      | sbobj.Groups(2).Signals(1).Name = 'v [km/h]'
      | sbobj.Groups(2).Signals(1).XData = [0 0.2 0.5 2 3 8 9 14 15]
      | sbobj.Groups(2).Signals(1).YData = [0 5 5 30 30 70 70 0 0]
      | sbobj.Groups(2).Signals(2).Name = 'grade[deg]'
      | sbobj.Groups(2).Signals(2).XData = [0 15]
      | sbobj.Groups(2).Signals(2).YData = [0 0]
      | sbobj.Groups(2).Signals(3).Name = 'vWind [m/s]'
      | sbobj.Groups(2).Signals(3).XData = [0 15]
      | sbobj.Groups(2).Signals(3).YData = [0 0]
      | sbobj.Groups(2).TimeRange = [0 15]
      | sbobj.Groups(3).Name = 'Group 3'
      | sbobj.Groups(3).Signals(1).Name = 'v [km/h]'
      | sbobj.Groups(3).Signals(1).XData = [0 0.25 9.5 10]
      | sbobj.Groups(3).Signals(1).YData = [40 40 80 80]
      | sbobj.Groups(3).Signals(2).Name = 'grade[deg]'
      | sbobj.Groups(3).Signals(2).XData = [0 10]
      | sbobj.Groups(3).Signals(2).YData = [0 0]
      | sbobj.Groups(3).Signals(3).Name = 'vWind [m/s]'
      | sbobj.Groups(3).Signals(3).XData = [0 10]
      | sbobj.Groups(3).Signals(3).YData = [0 0]
      | sbobj.Groups(4).Name = 'Group 4'
      | sbobj.Groups(4).Signals(1).Name = 'v [km/h]'
      | sbobj.Groups(4).Signals(1).XData = [0 4.7 10]
      | sbobj.Groups(4).Signals(1).YData = [0 30 30]
      | sbobj.Groups(4).Signals(2).Name = 'grade[deg]'
      | sbobj.Groups(4).Signals(2).XData = [0 5 9.5 10]
      | sbobj.Groups(4).Signals(2).YData = [0 0 40 40]
      | sbobj.Groups(4).Signals(3).Name = 'vWind [m/s]'
      | sbobj.Groups(4).Signals(3).XData = [0 5 9.5 10]
      | sbobj.Groups(4).Signals(3).YData = [0 0 40 40]
      | sbobj.Groups(5).Name = 'Group 5'
      | sbobj.Groups(5).Signals(1).Name = 'v [km/h]'
      | sbobj.Groups(5).Signals(1).XData = [0 1 2 5 7 10 12]
      | sbobj.Groups(5).Signals(1).YData = [0 7 7 30 30 7 7]
      | sbobj.Groups(5).Signals(2).Name = 'grade[deg]'
      | sbobj.Groups(5).Signals(2).XData = [0 12]
      | sbobj.Groups(5).Signals(2).YData = [0 0]
      | sbobj.Groups(5).Signals(3).Name = 'vWind [m/s]'
      | sbobj.Groups(5).Signals(3).XData = [0 12]
      | sbobj.Groups(5).Signals(3).YData = [0 0]
      | sbobj.Groups(5).TimeRange = [0 12]
      | sbobj.Groups(6).Name = 'Group 6'
      | sbobj.Groups(6).Signals(1).Name = 'v [km/h]'
      | sbobj.Groups(6).Signals(1).XData = [0 0.1 4 6 10 14 20 24.8 27.1 30]
      | sbobj.Groups(6).Signals(1).YData = [0 0 25 25 43 43 70 70 0 0]
      | sbobj.Groups(6).Signals(2).Name = 'grade[deg]'
      | sbobj.Groups(6).Signals(2).XData = [0 30]
      | sbobj.Groups(6).Signals(2).YData = [0 0]
      | sbobj.Groups(6).Signals(3).Name = 'vWind [m/s]'
      | sbobj.Groups(6).Signals(3).XData = [0 30]
      | sbobj.Groups(6).Signals(3).YData = [0 0]
      | sbobj.Groups(6).TimeRange = [0 30]
  v [km/h] : Outport  Tag=STV Outport  VectorParamsAs1DForOutWhenUnconnected=off
  grade[deg] : Outport  Tag=STV Outport  Port=2  VectorParamsAs1DForOutWhenUnconnected=off
  vWind [m/s] : Outport  Tag=STV Outport  Port=3  VectorParamsAs1DForOutWhenUnconnected=off
  wires:
  FromWs/1 -> Demux/1
  Demux/1 -> v [km/h]/1
  Demux/2 -> grade[deg]/1
  Demux/3 -> vWind [m/s]/1

== system vehicleVariantsLabel/control/Driver//Power Management/Driver//PI Anti Windup ==
  e : Inport
  u_sat : Inport  Port=2
  Constant : Constant  Value=0  SampleTime=-1
  Discrete PI Controller1 : eeDiscretePi/Discrete PI Controller  Kp=Kp_v  Ki=Ki_v  Kaw=100  x0=0  Ts=Tso
      settings: SourceProductBaseCode=PS
  Sum2 : Sum  Inputs=|-+
  u : Outport  VectorParamsAs1DForOutWhenUnconnected=off
  wires:
  e/1 -> Discrete PI Controller1/1
  Discrete PI Controller1/1 -> u/1, Sum2/1
  Sum2/1 -> Discrete PI Controller1/2
  Constant/1 -> Discrete PI Controller1/3
  u_sat/1 -> Sum2/2

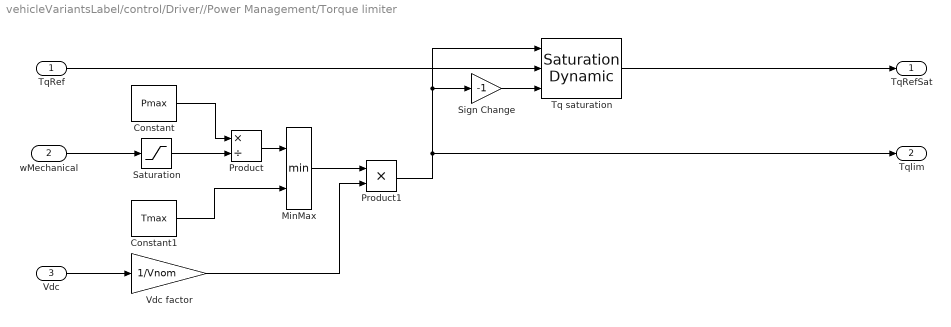
== system vehicleVariantsLabel/control/Driver//Power Management/Torque limiter ==
  TqRef : Inport
  wMechanical : Inport  Port=2
  Vdc : Inport  Port=3
  Constant : Constant  Value=Pmax  SampleTime=-1
  Constant1 : Constant  Value=Tmax  SampleTime=-1
  MinMax : MinMax  Inputs=2
  Product : Product  Inputs=*/
  Product1 : Product
  Saturation : Saturate  UpperLimit=inf  LowerLimit=Pmax/Tmax
  Sign Change : Gain  Gain=-1
  Tq saturation : simulink/Discontinuities/Saturation Dynamic  OutMin=[]  OutMax=[]  OutDataTypeStr=Inherit: Same as second input  OutDataType=fixdt(1, 16)  OutScaling=2^-10  DoSatur=off
  Vdc factor : Gain  Gain=1/Vnom
  TqRefSat : Outport  VectorParamsAs1DForOutWhenUnconnected=off
  Tqlim : Outport  Port=2  VectorParamsAs1DForOutWhenUnconnected=off
  wires:
  Vdc factor/1 -> Product1/2
  MinMax/1 -> Product1/1
  Sign Change/1 -> Tq saturation/3
  Saturation/1 -> Product/2
  Constant/1 -> Product/1
  Product/1 -> MinMax/1
  wMechanical/1 -> Saturation/1
  Constant1/1 -> MinMax/2
  Vdc/1 -> Vdc factor/1
  TqRef/1 -> Tq saturation/2
  Product1/1 -> Sign Change/1, Tq saturation/1, Tqlim/1
  Tq saturation/1 -> TqRefSat/1

== system vehicleVariantsLabel/control/Driver//Power Management/hybrid management ==
  MotTrqCmd : Inport
  Add : Sum  Inputs=-+
  Saturation : Saturate  UpperLimit=Inf  LowerLimit=recumax
  Saturation1 : Saturate  UpperLimit=0  LowerLimit=-inf
  EMotTrqCmd : Outport  VectorParamsAs1DForOutWhenUnconnected=off
  "FricBrakeTrqCmd " : Outport  Port=2  VectorParamsAs1DForOutWhenUnconnected=off
  wires:
  Add/1 -> Saturation1/1
  Saturation/1 -> EMotTrqCmd/1, Add/1
  Saturation1/1 -> "FricBrakeTrqCmd "/1
  MotTrqCmd/1 -> Saturation/1, Add/2

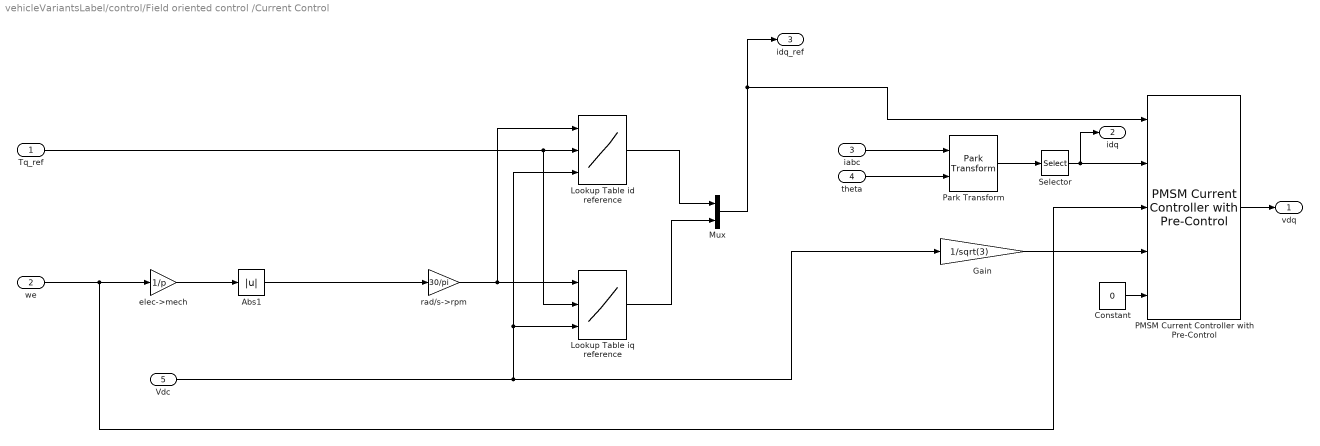
== system vehicleVariantsLabel/control/Field oriented control /Current Control ==
  Tq_ref : Inport
  we : Inport  Port=2
  iabc : Inport  Port=3
  theta : Inport  Port=4
  Vdc : Inport  Port=5
  Abs1 : Abs
  Constant : Constant  Value=0  SampleTime=Tsi
  Gain : Gain  Gain=1/sqrt(3)
  Lookup Table id reference : Lookup_n-D  NumberOfTableDimensions=3  BreakpointsForDimension1=RPM_VECT  BreakpointsForDimension2=TQ_VECT  BreakpointsForDimension3=VDC_VECT  Table=ID_MAP  InputSameDT=on
  Lookup Table iq reference : Lookup_n-D  NumberOfTableDimensions=3  BreakpointsForDimension1=RPM_VECT  BreakpointsForDimension2=TQ_VECT  BreakpointsForDimension3=VDC_VECT  Table=IQ_MAP  InputSameDT=on
  Mux : Mux  Inputs=2
  PMSM Current Controller with Pre-Control : eePmsmCurrentController/PMSM Current Controller with Pre-Control  Kp_id=Kp_id  Ki_id=Ki_id  Kaw_id=1  Kp_iq=Kp_iq  Ki_iq=Ki_iq  Kaw_iq=1  Ts=Tsi  Tsd=Tsi  AxisPrio=Q-axis  ActZC=off  ActFF=on  idVect=[-200, 0, 200]  iqVect=[-200, 0, 200]  LdMatrix=Ld * ones(3, 3)  LqMatrix=Lq * ones(3, 3)  psimMatrix=psim * ones(3, 3)
      settings: SourceProductBaseCode=PS
  Park Transform : eeTransforms/Park Transform  AxisAlignment=Q-axis  PowerInvariant=off
  Selector : Selector  InputPortWidth=3  IndexOptions=Index vector (dialog)  Indices=[1 2]  OutputSizes=1
  elec->mech : Gain  Gain=1/p
  rad/s->rpm : Gain  Gain=30/pi
  vdq : Outport  VectorParamsAs1DForOutWhenUnconnected=off
  idq : Outport  Port=2  VectorParamsAs1DForOutWhenUnconnected=off
  idq_ref : Outport  Port=3  VectorParamsAs1DForOutWhenUnconnected=off
  wires:
  Mux/1 -> idq_ref/1, PMSM Current Controller with Pre-Control/1
  Lookup Table id reference/1 -> Mux/1
  Lookup Table iq reference/1 -> Mux/2
  Vdc/1 -> Lookup Table id reference/3, Lookup Table iq reference/3, Gain/1
  rad/s->rpm/1 -> Lookup Table iq reference/1, Lookup Table id reference/1
  Abs1/1 -> rad/s->rpm/1
  elec->mech/1 -> Abs1/1
  we/1 -> elec->mech/1, PMSM Current Controller with Pre-Control/3
  Tq_ref/1 -> Lookup Table id reference/2, Lookup Table iq reference/2
  Gain/1 -> PMSM Current Controller with Pre-Control/4
  Park Transform/1 -> Selector/1
  Selector/1 -> PMSM Current Controller with Pre-Control/2, idq/1
  Constant/1 -> PMSM Current Controller with Pre-Control/5
  PMSM Current Controller with Pre-Control/1 -> vdq/1
  theta/1 -> Park Transform/2
  iabc/1 -> Park Transform/1

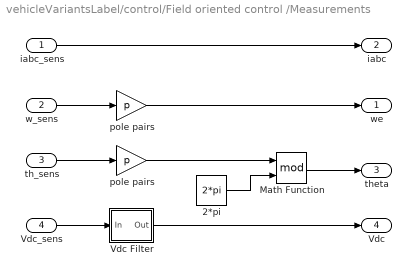
== system vehicleVariantsLabel/control/Field oriented control /Measurements ==
  iabc_sens : Inport
  w_sens : Inport  Port=2
  th_sens : Inport  Port=3
  Vdc_sens : Inport  Port=4
  2*pi : Constant  Value=2*pi  SampleTime=-1
  Math Function : Math  Operator=mod  SignedPower=on  SaturateOnIntegerOverflow=on
  Vdc Filter : Subsystem  mask(Discrete first-order filter (Low-pass)){T=0.005, Ts=1e-4}
      mask prompts: T "Time constant (s):"; Ts "Sample time (s):"
      mask help: This block implements a discrete low-pass filter. To calculate the coefficients, the block discretises a continuous low-pass filter using the Tustin method.
      mask init:
      | num = [ Ts/(2*T + Ts), Ts/(2*T + Ts)];
      | den = [ 1, -(2*T - Ts)/(2*T + Ts)];
  pole pairs : Gain  Gain=p
  "pole pairs " : Gain  Gain=p
  we : Outport  VectorParamsAs1DForOutWhenUnconnected=off
  iabc : Outport  Port=2  VectorParamsAs1DForOutWhenUnconnected=off
  theta : Outport  Port=3  VectorParamsAs1DForOutWhenUnconnected=off
  Vdc : Outport  Port=4  VectorParamsAs1DForOutWhenUnconnected=off
  wires:
  Vdc Filter/1(Out) -> Vdc/1
  Math Function/1 -> theta/1
  2*pi/1 -> Math Function/2
  "pole pairs "/1 -> Math Function/1
  iabc_sens/1 -> iabc/1
  w_sens/1 -> pole pairs/1
  th_sens/1 -> "pole pairs "/1
  Vdc_sens/1 -> Vdc Filter/1(In)
  pole pairs/1 -> we/1

== system vehicleVariantsLabel/control/Field oriented control /SVPWM ==
  Vabc : Inport
  vdc : Inport  Port=2
  MinMax SVM : Subsystem  VariantControl=Variant
  "PWM Generator (Three-phase, Two-level)" : eePwmGeneratorTwoLevel/PWM Generator (Three-phase, Two-level)  VariantControl=Variant1  PWMMode=Continuous PWM (CPWM)  CPWMMode=SVM: space vector modulation  DPWMMode=60 DPWM: 60 degree discontinuous PWM  fsw=fsw  Ts=Ts
      settings: SourceProductBaseCode=PS
  g : Outport  VectorParamsAs1DForOutWhenUnconnected=off
  ModWave : Outport  Port=2  VectorParamsAs1DForOutWhenUnconnected=off

== system vehicleVariantsLabel/plant/DC Source/DC ideal ==
  Constant : Constant  Value=0
  DC Voltage Source : fl_lib/Electrical/Electrical Sources/DC Voltage Source  v0=Vnom V
  Electrical Reference : fl_lib/Electrical/Electrical Elements/Electrical Reference
  + : PMIOPort  Side=Right
  - : PMIOPort  Port=2  Side=Right
  tag scope: SOC=global
  wires:
  Constant/1 -> [SOC]
  connections:
  DC Voltage Source/LConn1 -- +/RConn1
  DC Voltage Source/RConn1 -- Electrical Reference/LConn1 -- -/RConn1

== system vehicleVariantsLabel/plant/DC Source/battery ==
  Battery : ee_lib/Sources/Battery  Vnom=Vnom V  R1=1e-3 Ohm  prm_AH=1  AH=50 hr*A  V1=11.5 V  AH1=25 hr*A  prm_R2=1  R2=2000 Ohm  prm_dyn=1  Rp1=0.005 Ohm  tau1=30 s  Rp2=0.005 Ohm  tau2=30 s  Rp3=0.005 Ohm  tau3=30 s  Rp4=0.005 Ohm  tau4=30 s  Rp5=0.005 Ohm  tau5=30 s  prm_fade=1  N_fade=100  AH_fade=45 hr*A  R1_fade=2.02 Ohm  V1_fade=10.35 V  i_specify=off  i_priority=None  i=0 A  i_nominal_specify=off  i_nominal_unit=A  i_nominal_value=1  v_specify=off  v_priority=None  v=0 V  v_nominal_specify=off  v_nominal_unit=V  v_nominal_value=1  charge_specify=off  charge_priority=High  charge=50 hr*A  charge_nominal_specify=off  charge_nominal_unit=hr*A  charge_nominal_value=1  num_cycles_specify=off  num_cycles_priority=High  num_cycles=0  num_cycles_nominal_specify=off  num_cycles_nominal_unit=1  num_cycles_nominal_value=1  thermal_mass=30000 J/K  Tmeas=298.15 K  Vnom_T2=12 V  R1_T2=2.2 Ohm  V1_T2=11.4 V  R2_T2=2200 Ohm  Rp1_T2=0.005 Ohm  tau1_T2=30 s  Rp2_T2=0.005 Ohm  tau2_T2=30 s  Rp3_T2=0.005 Ohm  tau3_T2=30 s  Rp4_T2=0.005 Ohm  tau4_T2=30 s  Rp5_T2=0.005 Ohm  tau5_T2=30 s  Tmeas2=273.15 K  temperature_specify=off  temperature_priority=High  temperature=298.15 K  temperature_nominal_specify=off  temperature_nominal_unit=K  temperature_nominal_value=1
      settings: InternalSimscapePortConfiguration="{\"Bottom\":[],\"Left\":[{\"id\":\"p\",\"label\":\"+\",\"type\":\"foundation.electrical.electrical\"},{\"id\":\"q\",\"label\":\"q\",\"type\":\"output\"}],\"Right\":[{\"id\":\"n\",\"label\":\"-\",\"type\":\"foundation.electrical.electrical\"}],\"Top\":[]}"
  Electrical Reference : fl_lib/Electrical/Electrical Elements/Electrical Reference
  PS-Simulink Converter : nesl_utility/PS-Simulink Converter  PhysicalDomain=network_engine_domain  SubClassName=ps_output  LeftPortType=input  RightPortType=output  PseudoPeriodic=off  Frequencies=[]  Unit=hr*A  AffineConversion=off
  + : PMIOPort  Side=Right
  - : PMIOPort  Port=2  Side=Right
  tag scope: SOC=global
  wires:
  PS-Simulink Converter/1 -> [SOC]
  connections:
  Battery/LConn1 -- +/RConn1
  Battery/RConn1 -- Electrical Reference/LConn1 -- -/RConn1
  Battery/LConn2 -- PS-Simulink Converter/LConn1

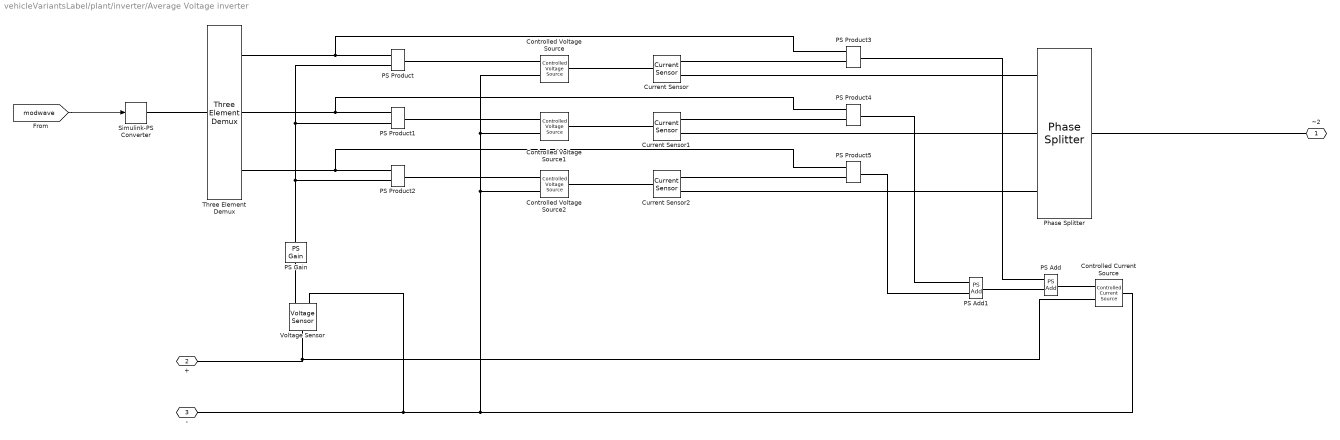
== system vehicleVariantsLabel/plant/inverter/Average Voltage inverter ==
  Controlled Current Source : fl_lib/Electrical/Electrical Sources/Controlled Current Source
  Controlled Voltage Source : fl_lib/Electrical/Electrical Sources/Controlled Voltage Source
  Controlled Voltage Source1 : fl_lib/Electrical/Electrical Sources/Controlled Voltage Source
  Controlled Voltage Source2 : fl_lib/Electrical/Electrical Sources/Controlled Voltage Source
  Current Sensor : fl_lib/Electrical/Electrical Sensors/Current Sensor
  Current Sensor1 : fl_lib/Electrical/Electrical Sensors/Current Sensor
  Current Sensor2 : fl_lib/Electrical/Electrical Sensors/Current Sensor
  PS Add : fl_lib/Physical Signals/Functions/PS Add
  PS Add1 : fl_lib/Physical Signals/Functions/PS Add
  PS Gain : fl_lib/Physical Signals/Functions/PS Gain  gain=0.5
  PS Product{,1..5} (6 alike) : fl_lib/Physical Signals/Functions/PS Product
  Phase Splitter : ee_lib/Connectors & References/Phase Splitter
      settings: SourceProductBaseCode=PS
  Simulink-PS Converter : nesl_utility/Simulink-PS Converter  PhysicalDomain=network_engine_domain  SubClassName=ps_input  LeftPortType=input  RightPortType=output  PseudoPeriodic=off  Frequencies=[]  NoiseDistribution=none  NoiseParameters=[]  Unit=1  AffineConversion=off  FilteringAndDerivatives=provide  SimscapeFilterOrder=1  InputFilterTimeConstant=0.001  UdotUserProvided=0
  Three Element Demux : ee_lib/Connectors & References/Three Element Demux
      settings: SourceProductBaseCode=PS  InternalSimscapePortConfiguration="{\"Bottom\":[],\"Left\":[{\"id\":\"abc\",\"label\":\"abc\",\"type\":\"input\"}],\"Right\":[{\"id\":\"a\",\"label\":\"a\",\"type\":\"output\"},{\"id\":\"b\",\"label\":\"b\",\"type\":\"output\"},{\"id\":\"c\",\"label\":\"c\",\"type\":\"output\"}],\"Top\":[]}"
  Voltage Sensor : fl_lib/Electrical/Electrical Sensors/Voltage Sensor
  ~2 : PMIOPort  Side=Right
  + : PMIOPort  Port=2  Side=Left
  - : PMIOPort  Port=3  Side=Left
  wires:
  [modwave] -> Simulink-PS Converter/1
  connections:
  ~2/RConn1 -- Phase Splitter/LConn1
  Three Element Demux/LConn1 -- Simulink-PS Converter/RConn1
  +/RConn1 -- Controlled Current Source/RConn2 -- Voltage Sensor/LConn1
  -/RConn1 -- Controlled Voltage Source/RConn2 -- Controlled Voltage Source1/RConn2 -- Controlled Voltage Source2/RConn2 -- Controlled Current Source/LConn1 -- Voltage Sensor/RConn2
  PS Gain/LConn1 -- Voltage Sensor/RConn1
  Controlled Voltage Source/RConn1 -- PS Product/RConn1
  Controlled Voltage Source1/RConn1 -- PS Product1/RConn1
  Controlled Voltage Source2/RConn1 -- PS Product2/RConn1
  Current Sensor/LConn1 -- Controlled Voltage Source/LConn1
  Current Sensor1/LConn1 -- Controlled Voltage Source1/LConn1
  Current Sensor2/LConn1 -- Controlled Voltage Source2/LConn1
  PS Product3/LConn2 -- Current Sensor/RConn1
  Current Sensor/RConn2 -- Phase Splitter/RConn1
  Current Sensor1/RConn2 -- Phase Splitter/RConn2
  Current Sensor2/RConn2 -- Phase Splitter/RConn3
  PS Product5/LConn2 -- Current Sensor2/RConn1
  Three Element Demux/RConn1 -- PS Product3/LConn1 -- PS Product/LConn1
  Three Element Demux/RConn2 -- PS Product4/LConn1 -- PS Product1/LConn1
  Three Element Demux/RConn3 -- PS Product5/LConn1 -- PS Product2/LConn1
  PS Gain/RConn1 -- PS Product1/LConn2 -- PS Product/LConn2 -- PS Product2/LConn2
  Current Sensor1/RConn1 -- PS Product4/LConn2
  PS Product3/RConn1 -- PS Add/LConn1
  PS Product4/RConn1 -- PS Add1/LConn1
  PS Product5/RConn1 -- PS Add1/LConn2
  PS Add1/RConn1 -- PS Add/LConn2
  Controlled Current Source/RConn1 -- PS Add/RConn1

== system vehicleVariantsLabel/plant/inverter/ideal inverter ==
  Converter1 : ee_lib/Semiconductors & Converters/Converters/Converter (Three-Phase)  device_type=3  Vf=0.8 V  Ron=0.055 Ohm  Rds=0.001 Ohm  Goff=1e-6 1/Ohm  Vth=0.5 V  Vgt=1 V  Vgt_off=-1 V  Ih=1 A  diode_param=2  diode_Vf=0.8 V  diode_Ron=0.001 Ohm  diode_Goff=1e-5 1/Ohm  diode_C=50 nF  diode_iRM=-235 A  diode_iF=300 A  diode_idot=-50 A/us  diode_trr_param=1  diode_trr_factor=3  diode_trr=15 us  diode_Qrr=1.5e+3 s*uA  snubber_type=0  Rs=0.1 Ohm  Cs=1e-7 F
      settings: SourceProductBaseCode=PS
  GateI1 : Subsystem
  + : PMIOPort  Side=Left
  - : PMIOPort  Port=2  Side=Left
  ~2 : PMIOPort  Port=3  Side=Right
  wires:
  [G] -> GateI1/1(S)
  connections:
  GateI1/RConn1 -- Converter1/LConn1
  Converter1/RConn1 -- +/RConn1
  Converter1/RConn2 -- -/RConn1
  Converter1/LConn2 -- ~2/RConn1

== system vehicleVariantsLabel/plant/mechanical load/load1 ==
  Ideal Torque Source : fl_lib/Mechanical/Mechanical Sources/Ideal Torque Source
  MRRef Load : fl_lib/Mechanical/Rotational Elements/Mechanical Rotational Reference
      settings: SourceProductName=Foundation Library
  Mechanical Translational Reference : fl_lib/Mechanical/Translational Elements/Mechanical Translational Reference
  PS Terminator : fl_lib/Physical Signals/Sinks/PS Terminator
      settings: SourceProductName=Foundation Library
  PS-Simulink Converter : nesl_utility/PS-Simulink Converter  PhysicalDomain=network_engine_domain  SubClassName=ps_output  LeftPortType=input  RightPortType=output  PseudoPeriodic=off  Frequencies=[]  Unit=m/s  AffineConversion=off
  Sensor : fl_lib/Mechanical/Mechanical Sensors/Ideal Translational Motion Sensor  offset=0 m
  Simulink-PS Converter1 : nesl_utility/Simulink-PS Converter  PhysicalDomain=network_engine_domain  SubClassName=ps_input  LeftPortType=input  RightPortType=output  PseudoPeriodic=off  Frequencies=[]  NoiseDistribution=none  NoiseParameters=[]  Unit=N*m  AffineConversion=off  FilteringAndDerivatives=zero  SimscapeFilterOrder=1  InputFilterTimeConstant=0.001  UdotUserProvided=1
  gear : fl_lib/Mechanical/Mechanisms/Gear Box  ratio=gveh  t_in_specify=off  t_in_priority=None  t_in=0 N*m  t_in_nominal_specify=off  t_in_nominal_unit=N*m  t_in_nominal_value=1  t_out_specify=off  t_out_priority=None  t_out=0 N*m  t_out_nominal_specify=off  t_out_nominal_unit=N*m  t_out_nominal_value=1
  inertia : fl_lib/Mechanical/Rotational Elements/Inertia  inertia=0.9 kg*m^2  w_specify=off  w_priority=High  w=0 rad/s  w_nominal_specify=off  w_nominal_unit=rad/s  w_nominal_value=1  t_specify=off  t_priority=None  t=0 N*m  t_nominal_specify=off  t_nominal_unit=N*m  t_nominal_value=1
  rotational-translational : fl_lib/Mechanical/Mechanisms/Wheel and Axle  R=rreifen m  or=1  t_specify=off  t_priority=None  t=0 N*m  t_nominal_specify=off  t_nominal_unit=N*m  t_nominal_value=1  f_specify=off  f_priority=None  f=0 N  f_nominal_specify=off  f_nominal_unit=N  f_nominal_value=1
  R : PMIOPort  Side=Left
  tag scope: v=global
  wires:
  PS-Simulink Converter/1 -> [v]
  [FricTrq_cmd] -> Simulink-PS Converter1/1
  connections:
  Sensor/RConn2 -- PS-Simulink Converter/LConn1
  Sensor/RConn1 -- Mechanical Translational Reference/LConn1
  rotational-translational/LConn1 -- gear/RConn1
  PS Terminator/LConn1 -- Sensor/RConn3
  rotational-translational/RConn1 -- Sensor/LConn1
  MRRef Load/LConn1 -- Ideal Torque Source/RConn2
  Simulink-PS Converter1/RConn1 -- Ideal Torque Source/RConn1
  gear/LConn1 -- inertia/LConn1 -- R/RConn1 -- Ideal Torque Source/LConn1

== system vehicleVariantsLabel/plant/mechanical load/load2 ==
  Ideal Torque Source : fl_lib/Mechanical/Mechanical Sources/Ideal Torque Source
  MRRef Load : fl_lib/Mechanical/Rotational Elements/Mechanical Rotational Reference
      settings: SourceProductName=Foundation Library
  Mechanical Translational Reference : fl_lib/Mechanical/Translational Elements/Mechanical Translational Reference
  PS Terminator : fl_lib/Physical Signals/Sinks/PS Terminator
      settings: SourceProductName=Foundation Library
  PS-Simulink Converter : nesl_utility/PS-Simulink Converter  PhysicalDomain=network_engine_domain  SubClassName=ps_output  LeftPortType=input  RightPortType=output  PseudoPeriodic=off  Frequencies=[]  Unit=m/s  AffineConversion=off
  Sensor : fl_lib/Mechanical/Mechanical Sensors/Ideal Translational Motion Sensor  offset=0 m
  Simulink-PS Converter1 : nesl_utility/Simulink-PS Converter  PhysicalDomain=network_engine_domain  SubClassName=ps_input  LeftPortType=input  RightPortType=output  PseudoPeriodic=off  Frequencies=[]  NoiseDistribution=none  NoiseParameters=[]  Unit=N*m  AffineConversion=off  FilteringAndDerivatives=zero  SimscapeFilterOrder=1  InputFilterTimeConstant=0.001  UdotUserProvided=1
  gear : fl_lib/Mechanical/Mechanisms/Gear Box  ratio=gveh  t_in_specify=off  t_in_priority=None  t_in=0 N*m  t_in_nominal_specify=off  t_in_nominal_unit=N*m  t_in_nominal_value=1  t_out_specify=off  t_out_priority=None  t_out=0 N*m  t_out_nominal_specify=off  t_out_nominal_unit=N*m  t_out_nominal_value=1
  inertia : fl_lib/Mechanical/Rotational Elements/Inertia  inertia=0.9 kg*m^2  w_specify=off  w_priority=High  w=0 rad/s  w_nominal_specify=off  w_nominal_unit=rad/s  w_nominal_value=1  t_specify=off  t_priority=None  t=0 N*m  t_nominal_specify=off  t_nominal_unit=N*m  t_nominal_value=1
  rotational-translational : fl_lib/Mechanical/Mechanisms/Wheel and Axle  R=rreifen m  or=1  t_specify=off  t_priority=None  t=0 N*m  t_nominal_specify=off  t_nominal_unit=N*m  t_nominal_value=1  f_specify=off  f_priority=None  f=0 N  f_nominal_specify=off  f_nominal_unit=N  f_nominal_value=1
  R : PMIOPort  Side=Left
  tag scope: v=global
  wires:
  [FricTrq_cmd] -> Simulink-PS Converter1/1
  PS-Simulink Converter/1 -> [v]
  connections:
  Ideal Torque Source/LConn1 -- R/RConn1 -- gear/LConn1 -- inertia/LConn1
  Simulink-PS Converter1/RConn1 -- Ideal Torque Source/RConn1
  MRRef Load/LConn1 -- Ideal Torque Source/RConn2
  rotational-translational/RConn1 -- Sensor/LConn1
  PS Terminator/LConn1 -- Sensor/RConn3
  rotational-translational/LConn1 -- gear/RConn1
  Sensor/RConn1 -- Mechanical Translational Reference/LConn1
  Sensor/RConn2 -- PS-Simulink Converter/LConn1

== system vehicleVariantsLabel/control/Field oriented control /Measurements/Vdc Filter ==
  In : Inport
  Discrete Transfer Fcn : DiscreteTransferFcn  Numerator=num  Denominator=den
  Out : Outport  VectorParamsAs1DForOutWhenUnconnected=off
  wires:
  In/1 -> Discrete Transfer Fcn/1
  Discrete Transfer Fcn/1 -> Out/1

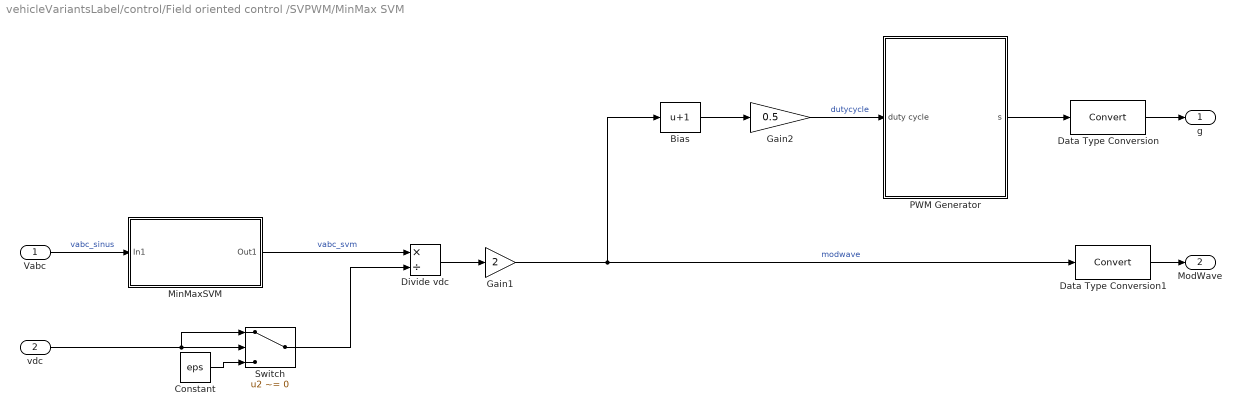
== system vehicleVariantsLabel/control/Field oriented control /SVPWM/MinMax SVM ==
  Vabc : Inport
  vdc : Inport  Port=2
  Bias : Bias  Bias=1
  Constant : Constant  Value=eps
  Data Type Conversion : DataTypeConversion
  Data Type Conversion1 : DataTypeConversion
  Divide vdc : Product  Inputs=*/
  Gain1 : Gain  Gain=2
  Gain2 : Gain  Gain=0.5
  MinMaxSVM : Subsystem
  PWM Generator : Subsystem
  Switch : Switch  Criteria=u2 ~= 0
  g : Outport  VectorParamsAs1DForOutWhenUnconnected=off
  ModWave : Outport  Port=2  VectorParamsAs1DForOutWhenUnconnected=off
  wires:
  Divide vdc/1 -> Gain1/1
  Gain1/1 -> Data Type Conversion1/1, Bias/1  "modwave"
  Vabc/1 -> MinMaxSVM/1(In1)  "vabc_sinus"
  MinMaxSVM/1(Out1) -> Divide vdc/1  "vabc_svm"
  Bias/1 -> Gain2/1
  Gain2/1 -> PWM Generator/1(duty cycle)  "dutycycle"
  PWM Generator/1(s) -> Data Type Conversion/1
  Data Type Conversion/1 -> g/1
  Data Type Conversion1/1 -> ModWave/1
  Switch/1 -> Divide vdc/2
  vdc/1 -> Switch/1, Switch/2
  Constant/1 -> Switch/3

== system vehicleVariantsLabel/plant/inverter/ideal inverter/GateI1 ==
  S : Inport
  Demux : Demux  Outputs=6
  Simulink-PS Converter{1..6} (6 alike) : nesl_utility/Simulink-PS Converter  PhysicalDomain=network_engine_domain  SubClassName=ps_input  LeftPortType=input  RightPortType=output  PseudoPeriodic=off  Frequencies=[]  NoiseDistribution=none  NoiseParameters=[]  Unit=1  AffineConversion=off  FilteringAndDerivatives=zero  SimscapeFilterOrder=1  InputFilterTimeConstant=0.001  UdotUserProvided=1
  Six-Pulse Gate Multiplexer : ee_lib/Semiconductors & Converters/Converters/Six-Pulse Gate Multiplexer  R=0 Ohm
      settings: SourceProductBaseCode=PS  InternalSimscapePortConfiguration="{\"Bottom\":[],\"Left\":[{\"id\":\"GaH\",\"label\":\"Ga(H)\",\"type\":\"input\"},{\"id\":\"GaL\",\"label\":\"Ga(L)\",\"type\":\"input\"},{\"id\":\"GbH\",\"label\":\"Gb(H)\",\"type\":\"input\"},{\"id\":\"GbL\",\"label\":\"Gb(L)\",\"type\":\"input\"},{\"id\":\"GcH\",\"label\":\"Gc(H)\",\"type\":\"input\"},{\"id\":\"GcL\",\"label\":\"Gc(L)\",\"type\":\"input\"}],\"Right\":[{\"id\":\"p\",\"label\":\"G\",\"type\":\"foundation.electrical.twelve_phase\"}],\"Top\":[]}"
  G : PMIOPort  Side=Right
  wires:
  Demux/3 -> Simulink-PS Converter3/1
  Demux/6 -> Simulink-PS Converter6/1
  Demux/5 -> Simulink-PS Converter5/1
  S/1 -> Demux/1
  Demux/2 -> Simulink-PS Converter2/1
  Demux/1 -> Simulink-PS Converter1/1
  Demux/4 -> Simulink-PS Converter4/1
  connections:
  Six-Pulse Gate Multiplexer/RConn1 -- G/RConn1
  Six-Pulse Gate Multiplexer/LConn1 -- Simulink-PS Converter1/RConn1
  Simulink-PS Converter5/RConn1 -- Six-Pulse Gate Multiplexer/LConn5
  Simulink-PS Converter6/RConn1 -- Six-Pulse Gate Multiplexer/LConn6
  Simulink-PS Converter3/RConn1 -- Six-Pulse Gate Multiplexer/LConn3
  Simulink-PS Converter2/RConn1 -- Six-Pulse Gate Multiplexer/LConn2
  Simulink-PS Converter4/RConn1 -- Six-Pulse Gate Multiplexer/LConn4

== system vehicleVariantsLabel/control/Field oriented control /SVPWM/MinMax SVM/MinMaxSVM ==
  In1 : Inport
  Add : Sum
  Add1 : Sum  Inputs=+-
  Gain : Gain  Gain=0.5
  Max : MinMax  Function=max
  Max1 : MinMax
  Rate Transition1 : RateTransition  OutPortSampleTime=Ts
  Out1 : Outport  VectorParamsAs1DForOutWhenUnconnected=off
  wires:
  Add1/1 -> Out1/1
  Max1/1 -> Add/2
  In1/1 -> Rate Transition1/1
  Add/1 -> Gain/1
  Rate Transition1/1 -> Max1/1, Add1/1, Max/1
  Gain/1 -> Add1/2
  Max/1 -> Add/1

== system vehicleVariantsLabel/control/Field oriented control /SVPWM/MinMax SVM/PWM Generator ==
  duty cycle : Inport
  Logical Operator3 : Logic  Operator=NOT  AllPortsSameDT=off  OutDataTypeStr=boolean
  Mux : Mux  Inputs=2
  Relational Operator : RelationalOperator  Operator=<  OutDataTypeStr=boolean  RndMeth=Nearest
  Selector : Selector  InputPortWidth=6  IndexOptions=Index vector (dialog)  Indices=[1 4 2 5 3 6]  OutputSizes=1
  sawtooth : Subsystem  mask{fsw=fsw, upv=1, lowv=0}
      mask prompts: fsw "Switching frequency"; upv "Upper Threshold"; lowv "Lower Threshold"
  s : Outport  VectorParamsAs1DForOutWhenUnconnected=off
  wires:
  Relational Operator/1 -> Logical Operator3/1, Mux/1
  Logical Operator3/1 -> Mux/2
  Mux/1 -> Selector/1
  Selector/1 -> s/1
  duty cycle/1 -> Relational Operator/2
  sawtooth/1(Out1) -> Relational Operator/1
